simulink library "dsrc_handler"  (Simulink 8.2)
settings: Solver=ode1  StartTime=0.0  StopTime=Inf  FixedStep=0.001  RelTol=1e-3
PostLoadFcn:
  | , if any(exist('dsrtsu_mdlpostloadfcn', 'file') == [2, 3, 6]), try dsrtsu_mdlpostloadfcn('Execute', bdroot); catch fprintf('Error in PostLoadFcn (dsrtsu_mdlpostloadfcn) for model "%s":\n %s\n', bdroot, lasterr); end, end,
libraries: ParsingLibrary x1
settings Model: DSRTSU_INTERNAL_RTI_VER=440  DSRTSU_INTERNAL_RTI_TYPE=rti1401  DSRTSU_INTERNAL_RTIFPGA=30  Creator=leidos  LastModifiedBy=Admin

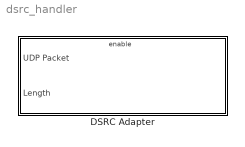
== system dsrc_handler ==
  DSRC Adapter : Subsystem

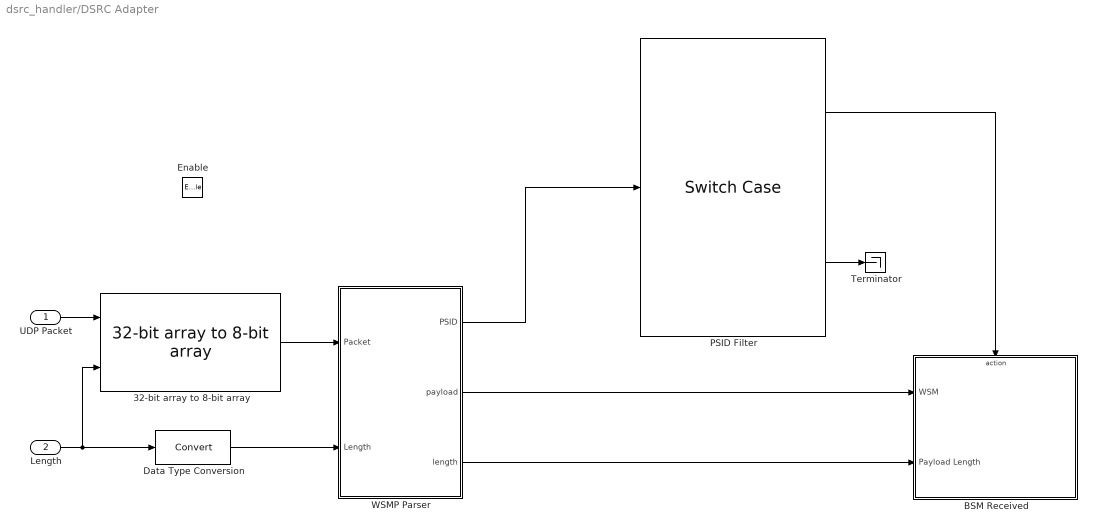
== system dsrc_handler/DSRC Adapter ==
  UDP Packet : Inport  OutDataTypeStr=uint32  PortDimensions=368
  Length : Inport  Port=2
  Enable : EnablePort
  32-bit array to 8-bit array : ParsingLibrary/32-bit array to 8-bit array
  BSM Received : Subsystem  TreatAsAtomicUnit=on
  Data Type Conversion : DataTypeConversion
  PSID Filter : SwitchCase  CaseConditions={2}
  Terminator : Terminator
  WSMP Parser : MATLAB Function  TreatAsAtomicUnit=on
  wires:
  32-bit array to 8-bit array/1 -> WSMP Parser/1(Packet)
  Length/1 -> 32-bit array to 8-bit array/2, Data Type Conversion/1
  PSID Filter/2 -> Terminator/1
  PSID Filter/1 -> BSM Received/Action
  WSMP Parser/3(length) -> BSM Received/2(Payload Length)
  UDP Packet/1 -> 32-bit array to 8-bit array/1
  WSMP Parser/2(payload) -> BSM Received/1(WSM)
  WSMP Parser/1(PSID) -> PSID Filter/1
  Data Type Conversion/1 -> WSMP Parser/2(Length)

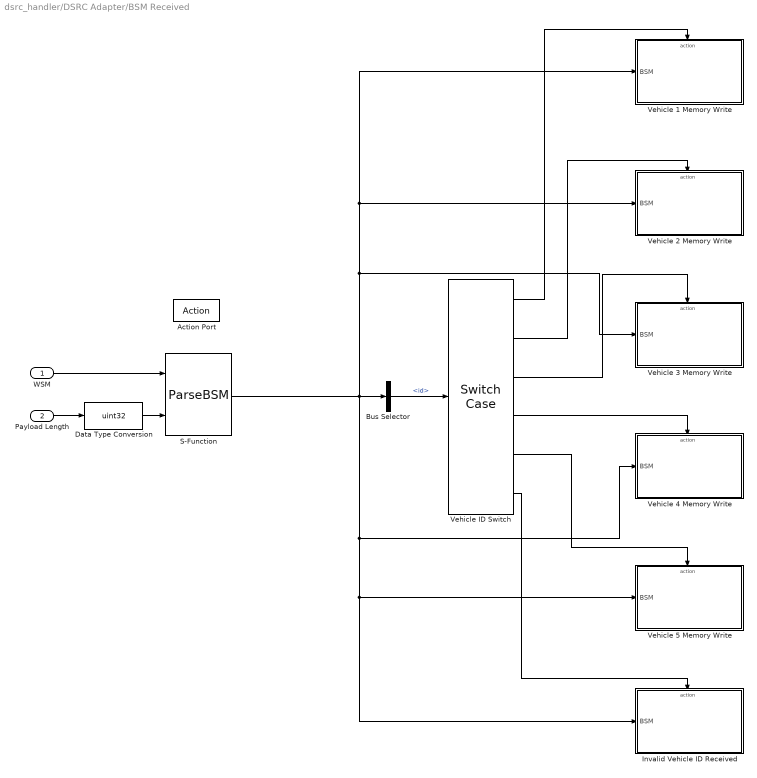
== system dsrc_handler/DSRC Adapter/BSM Received ==
  WSM : Inport  OutDataTypeStr=uint8  PortDimensions=1472
  Payload Length : Inport  Port=2
  Action Port : ActionPort
  Bus Selector : BusSelector  OutputSignals=id
  Data Type Conversion : DataTypeConversion  OutDataTypeStr=uint32
  Invalid Vehicle ID Received : Subsystem  TreatAsAtomicUnit=on
  S-Function : S-Function  FunctionName=ParseBSM  SFunctionModules='ParseBSM_wrapper bsm_parser der_decoder'  EnableBusSupport=off
  Vehicle 1 Memory Write : Subsystem  TreatAsAtomicUnit=on
  Vehicle 2 Memory Write : Subsystem  TreatAsAtomicUnit=on
  Vehicle 3 Memory Write : Subsystem  TreatAsAtomicUnit=on
  Vehicle 4 Memory Write : Subsystem  TreatAsAtomicUnit=on
  Vehicle 5 Memory Write : Subsystem  TreatAsAtomicUnit=on
  Vehicle ID Switch : SwitchCase  CaseConditions={96,97,98,99,100}
  wires:
  Bus Selector/1 -> Vehicle ID Switch/1  "<id>"
  Payload Length/1 -> Data Type Conversion/1
  WSM/1 -> S-Function/1
  Vehicle ID Switch/3 -> Vehicle 3 Memory Write/Action
  Vehicle ID Switch/5 -> Vehicle 5 Memory Write/Action
  Vehicle ID Switch/6 -> Invalid Vehicle ID Received/Action
  Vehicle ID Switch/4 -> Vehicle 4 Memory Write/Action
  Vehicle ID Switch/2 -> Vehicle 2 Memory Write/Action
  Vehicle ID Switch/1 -> Vehicle 1 Memory Write/Action
  S-Function/1 -> Invalid Vehicle ID Received/1(BSM), Vehicle 5 Memory Write/1(BSM), Vehicle 4 Memory Write/1(BSM), Bus Selector/1, Vehicle 1 Memory Write/1(BSM), Vehicle 2 Memory Write/1(BSM), Vehicle 3 Memory Write/1(BSM)
  Data Type Conversion/1 -> S-Function/2

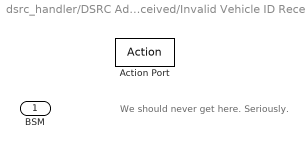
== system dsrc_handler/DSRC Adapter/BSM Received/Invalid Vehicle ID Received ==
  note: We should never get here. Seriously.
  BSM : Inport
  Action Port : ActionPort

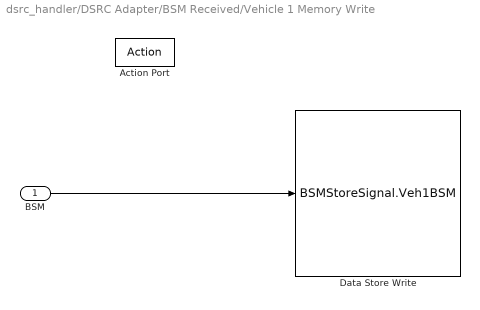
== system dsrc_handler/DSRC Adapter/BSM Received/Vehicle 1 Memory Write ==
  BSM : Inport
  Action Port : ActionPort
  Data Store Write : DataStoreWrite  DataStoreName=BSMStoreSignal  DataStoreElements=BSMStoreSignal.Veh1BSM
  wires:
  BSM/1 -> Data Store Write/1

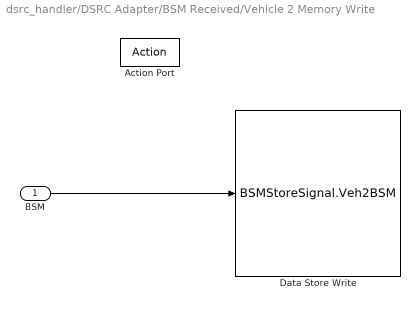
== system dsrc_handler/DSRC Adapter/BSM Received/Vehicle 2 Memory Write ==
  BSM : Inport
  Action Port : ActionPort
  Data Store Write : DataStoreWrite  DataStoreName=BSMStoreSignal  DataStoreElements=BSMStoreSignal.Veh2BSM
  wires:
  BSM/1 -> Data Store Write/1

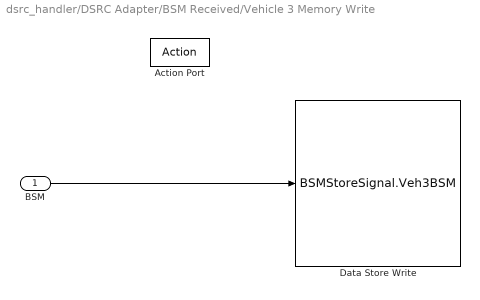
== system dsrc_handler/DSRC Adapter/BSM Received/Vehicle 3 Memory Write ==
  BSM : Inport
  Action Port : ActionPort
  Data Store Write : DataStoreWrite  DataStoreName=BSMStoreSignal  DataStoreElements=BSMStoreSignal.Veh3BSM
  wires:
  BSM/1 -> Data Store Write/1

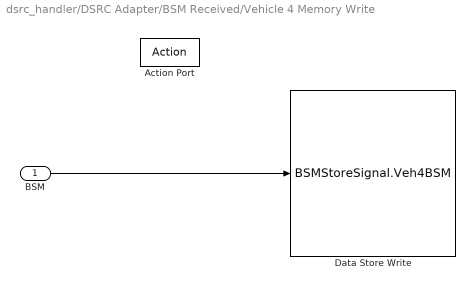
== system dsrc_handler/DSRC Adapter/BSM Received/Vehicle 4 Memory Write ==
  BSM : Inport
  Action Port : ActionPort
  Data Store Write : DataStoreWrite  DataStoreName=BSMStoreSignal  DataStoreElements=BSMStoreSignal.Veh4BSM
  wires:
  BSM/1 -> Data Store Write/1

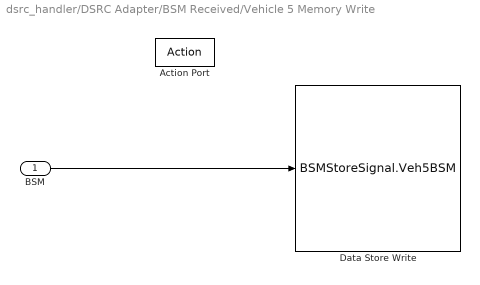
== system dsrc_handler/DSRC Adapter/BSM Received/Vehicle 5 Memory Write ==
  BSM : Inport
  Action Port : ActionPort
  Data Store Write : DataStoreWrite  DataStoreName=BSMStoreSignal  DataStoreElements=BSMStoreSignal.Veh5BSM
  wires:
  BSM/1 -> Data Store Write/1

== matlab function DSRC Adapter/WSMP Parser ==
  data: Packet input uint8; PSID output double; payload output uint8 size=1472; length output uint32; Length input uint32
function [PSID, payload,             length] = fcn(Packet, Length)
%#codegen

% Mock block, just to layout diagram
PSID = 2;

% TODO: Parse msgID out of WSM packet

payload = transpose(Packet);
length = Length;
